simulink model "inverse_controller"  (R2020a)
settings: Solver=FixedStepAuto  StartTime=0.0  StopTime=700  FixedStep=0.01  RelTol=1e-3
undefined symbols (not defined in the file): C, W
libraries: cstblocks x1, simulink x1
settings Model: Creator=Alejo  LastModifiedBy=elkin
settings DataIOCC: ReturnWorkspaceOutputs=off
settings DebuggingCC: ArithmeticOperatorsInVariantConditions=warning
settings SFSimCC: CustomCodeUndefinedFunction=UseInterfaceOnly

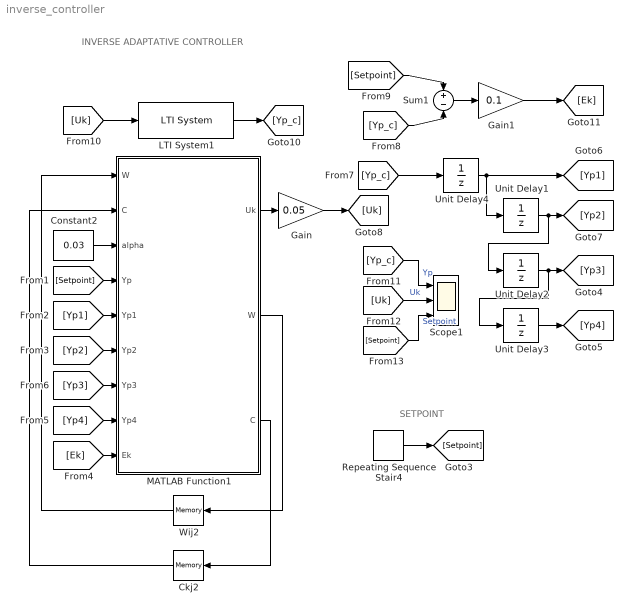
== system inverse_controller ==
  note: SETPOINT
  note: INVERSE ADAPTATIVE CONTROLLER
  Ckj2 : Memory  InitialCondition=C
  Constant2 : Constant  Value=0.03
  Gain : Gain  Gain=0.05
  Gain1 : Gain  Gain=0.1
  LTI System1 : cstblocks/LTI System  sys=servomotor  IC=[]
  MATLAB Function1 : MATLAB Function  TreatAsAtomicUnit=on
  Repeating Sequence Stair4 : simulink/Sources/Repeating Sequence Stair  OutValues=[0.4 0.2 0.1 0.4 0.3 0.4 0.5].'  tsamp=50  OutMin=[]  OutMax=[]  OutDataTypeStr=double  OutputDataTypeScalingMode=double  OutDataType=fixdt(0,8)  ConRadixGroup=Best Precision: Vector-wise  OutScaling=2^-12
  Scope1 : Scope  NumInputPorts=3
  Sum1 : Sum  Inputs=+-
  Unit Delay{1..4} (4 alike) : UnitDelay  SampleTime=-1  HasFrameUpgradeWarning=on
  Wij2 : Memory  InitialCondition=W
  wires:
  Gain/1 -> [Uk]
  Unit Delay1/1 -> Unit Delay2/1, [Yp2]
  [Yp4] -> MATLAB Function1/8(Yp4)
  MATLAB Function1/3(C) -> Ckj2/1
  MATLAB Function1/1(Uk) -> Gain/1
  Unit Delay4/1 -> [Yp1], Unit Delay1/1
  Unit Delay2/1 -> Unit Delay3/1, [Yp3]
  [Yp_c] -> Unit Delay4/1
  [Yp3] -> MATLAB Function1/7(Yp3)
  [Yp1] -> MATLAB Function1/5(Yp1)
  Constant2/1 -> MATLAB Function1/3(alpha)
  MATLAB Function1/2(W) -> Wij2/1
  [Yp2] -> MATLAB Function1/6(Yp2)
  [Ek] -> MATLAB Function1/9(Ek)
  Ckj2/1 -> MATLAB Function1/2("C ")
  [Setpoint] -> MATLAB Function1/4(Yp)
  Unit Delay3/1 -> [Yp4]
  Repeating Sequence Stair4/1 -> [Setpoint]
  Wij2/1 -> MATLAB Function1/1("W ")
  LTI System1/1 -> [Yp_c]
  [Setpoint] -> Sum1/1
  [Yp_c] -> Sum1/2
  [Uk] -> LTI System1/1
  [Yp_c] -> Scope1/1  "Yp"
  [Uk] -> Scope1/2  "Uk"
  [Setpoint] -> Scope1/3  "Setpoint"
  Sum1/1 -> Gain1/1
  Gain1/1 -> [Ek]

== matlab function inverse_controller/MATLAB Function1 ==
  data: W input; Uk output; C input; alpha input; Yp input; Yp1 input; Yp2 input; Yp3 input; Yp4 input; Ek input; W output; C output
function [Uk, W, C] = fcn(W, C, alpha, Yp, Yp1, Yp2, Yp3, Yp4, Ek)
    % Define input vector
    X = [Yp Yp1 Yp2 Yp3 Yp4];
    
    % Calculate Aj in the hidden layer
    Aj = W*X';
    
    % Activation function of the hidden layer
    H = tanh(Aj);
    
    % Calculate Ak in the output layer
    Ak = C'*H;
    
    % Activation function of the output layer
    Uk = Ak;
    
    % Update C matrix
    C = C + alpha*Ek*H;
    
    % Update W matrix
    Hd = sech(Aj).^2;
    W = W + alpha*Ek*(C.*Hd)*X;
